simulink model "Uppgift8"  (R2021a)
settings: Solver=VariableStepAuto  StartTime=0.0  StopTime=100  RelTol=1e-3
libraries: simulink_extras x1
settings Model: Creator=emiwi425  LastModifiedBy=emiwi425

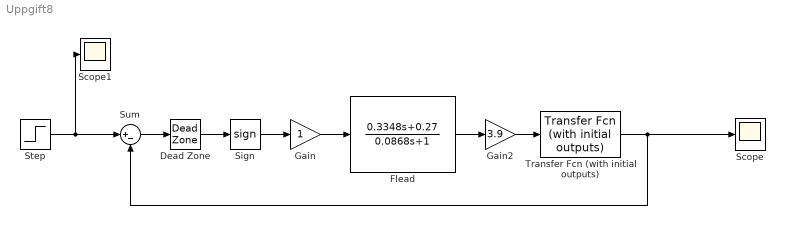
== system Uppgift8 ==
  Dead Zone : DeadZone  LowerValue=-0.2  UpperValue=0.2  SaturateOnIntegerOverflow=on
  Flead : TransferFcn  Numerator=[0.3348 0.27]  Denominator=[0.0868 1]
  Gain : Gain
  Gain2 : Gain  Gain=3.9
  Scope : Scope
  Scope1 : Scope
  Sign : Signum
  Step : Step  Time=10  After=2  SampleTime=0
  Sum : Sum  Inputs=|+-
  Transfer Fcn (with initial outputs) : simulink_extras/Additional Linear/Transfer Fcn (with initial outputs)  N=[45]  D="[1  10 9 0]"  Y0=0  U0=0
  wires:
  Sum/1 -> Dead Zone/1
  Dead Zone/1 -> Sign/1
  Sign/1 -> Gain/1
  Transfer Fcn (with initial outputs)/1 -> Sum/2, Scope/1
  Step/1 -> Scope1/1, Sum/1
  Gain/1 -> Flead/1
  Gain2/1 -> Transfer Fcn (with initial outputs)/1
  Flead/1 -> Gain2/1
